simulink model "lsys2"  (R2020b)
settings: Solver=VariableStepAuto  StartTime=0.0  StopTime=10.0  RelTol=1e-3
settings Model: Creator=반달  LastModifiedBy=반달

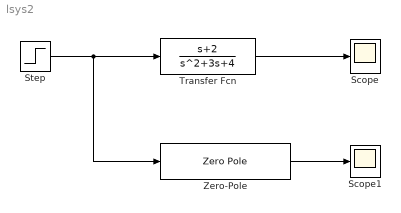
== system lsys2 ==
  Scope : Scope
  Scope1 : Scope
  Step : Step  Time=0  SampleTime=0
  Transfer Fcn : TransferFcn  Numerator=[1 2]  Denominator=[1 3 4]
  Zero-Pole : ZeroPole  Zeros=[1 3]  Poles=[-1 -2 -3]  Gain=2
  wires:
  Step/1 -> Zero-Pole/1, Transfer Fcn/1
  Zero-Pole/1 -> Scope1/1
  Transfer Fcn/1 -> Scope/1
